simulink model "simulacao"  (R2021a)
settings: Solver=VariableStepAuto  StartTime=0.0  StopTime=15  RelTol=1e-3
libraries: simulink x1
settings Model: Creator=gabriel  LastModifiedBy=gabriel

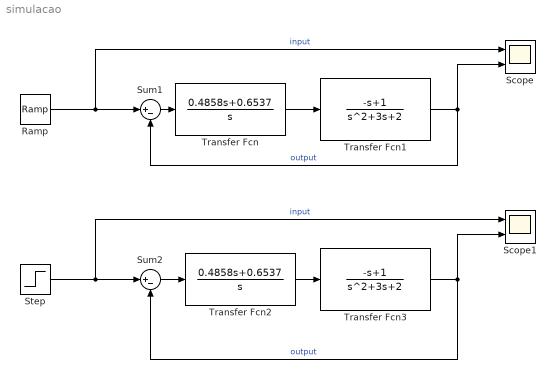
== system simulacao ==
  Ramp : simulink/Sources/Ramp  slope=1  start=0  InitialOutput=0
  Scope : Scope  NumInputPorts=2
  Scope1 : Scope  NumInputPorts=2
  Step : Step  SampleTime=0
  Sum1 : Sum  Inputs=|+-
  Sum2 : Sum  Inputs=|+-
  Transfer Fcn : TransferFcn  Numerator=[0.4858 0.6537]  Denominator=[1 0]
  Transfer Fcn1 : TransferFcn  Numerator=[-1 1]  Denominator=[1 3 2]
  Transfer Fcn2 : TransferFcn  Numerator=[0.4858 0.6537]  Denominator=[1 0]
  Transfer Fcn3 : TransferFcn  Numerator=[-1 1]  Denominator=[1 3 2]
  wires:
  Transfer Fcn/1 -> Transfer Fcn1/1
  Transfer Fcn1/1 -> Scope/2, Sum1/2  "output"
  Sum1/1 -> Transfer Fcn/1
  Ramp/1 -> Sum1/1, Scope/1  "input"
  Transfer Fcn3/1 -> Sum2/2, Scope1/2  "output"
  Transfer Fcn2/1 -> Transfer Fcn3/1
  Step/1 -> Sum2/1, Scope1/1  "input"
  Sum2/1 -> Transfer Fcn2/1
